simulink model "Ex_xyz"  (R2017b)
settings: Solver=VariableStepAuto  StartTime=0.0  StopTime=1  RelTol=1e-3
settings Model: Creator=81068  LastModifiedBy=81068

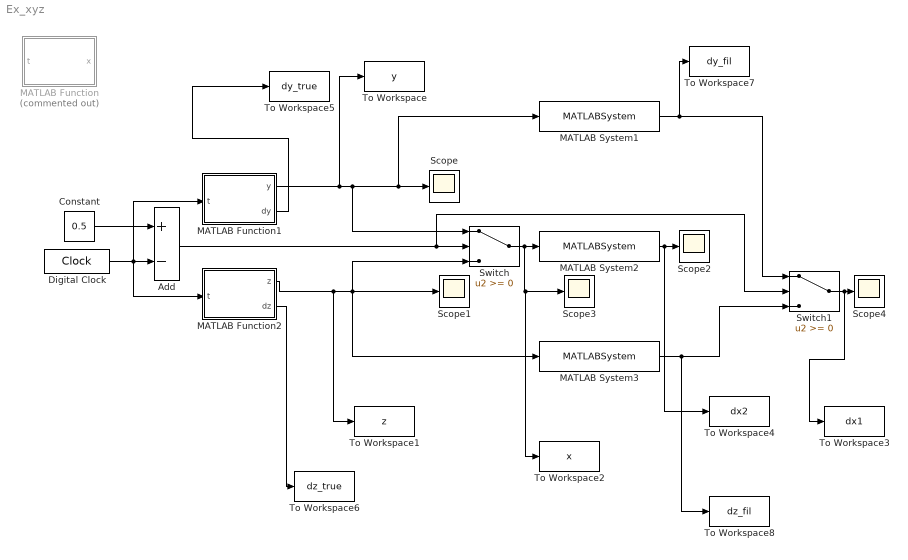
== system Ex_xyz ==
  Add : Sum  Inputs=+-
  Constant : Constant  Value=0.5
  Digital Clock : DigitalClock  SampleTime=1/2000
  MATLAB Function : MATLAB Function  Commented=on  TreatAsAtomicUnit=on
  MATLAB Function1 : MATLAB Function  TreatAsAtomicUnit=on
  MATLAB Function2 : MATLAB Function  TreatAsAtomicUnit=on
  MATLAB System1 : MATLABSystem  System=PolyRegressionFilter  sample_time=1/2000  history_length=10  dop=1  signal_dim=1  delay=RegressionDelay  SimulateUsing=Code generation
      mask Type: PolyRegressionFilter
      mask Display:
      | disp('PolyRegressionFilter');
      | port_label('input',1,'q');
      | port_label('output',1,'dq');
  MATLAB System2 : MATLABSystem  System=PolyRegressionFilter  sample_time=1/2000  history_length=10  dop=1  signal_dim=1  delay=RegressionDelay  SimulateUsing=Code generation
      mask Type: PolyRegressionFilter
      mask Display:
      | disp('PolyRegressionFilter');
      | port_label('input',1,'q');
      | port_label('output',1,'dq');
  MATLAB System3 : MATLABSystem  System=PolyRegressionFilter  sample_time=1/2000  history_length=10  dop=1  signal_dim=1  delay=RegressionDelay  SimulateUsing=Code generation
      mask Type: PolyRegressionFilter
      mask Display:
      | disp('PolyRegressionFilter');
      | port_label('input',1,'q');
      | port_label('output',1,'dq');
  Scope{,1..4} (5 alike) : Scope
  Switch : Switch
  Switch1 : Switch
  To Workspace : ToWorkspace  VariableName=y  SaveFormat=Timeseries  SampleTime=-1
  To Workspace1 : ToWorkspace  VariableName=z  SaveFormat=Timeseries  SampleTime=-1
  To Workspace2 : ToWorkspace  VariableName=x  SaveFormat=Timeseries  SampleTime=-1
  To Workspace3 : ToWorkspace  VariableName=dx1  SaveFormat=Timeseries  SampleTime=-1
  To Workspace4 : ToWorkspace  VariableName=dx2  SaveFormat=Timeseries  SampleTime=-1
  To Workspace5 : ToWorkspace  VariableName=dy_true  SaveFormat=Timeseries  SampleTime=-1
  To Workspace6 : ToWorkspace  VariableName=dz_true  SaveFormat=Timeseries  SampleTime=-1
  To Workspace7 : ToWorkspace  VariableName=dy_fil  SaveFormat=Timeseries  SampleTime=-1
  To Workspace8 : ToWorkspace  VariableName=dz_fil  SaveFormat=Timeseries  SampleTime=-1
  wires:
  Constant/1 -> Add/1
  Digital Clock/1 -> MATLAB Function2/1(t), MATLAB Function1/1(t), Add/2
  Add/1 -> Switch1/2, Switch/2
  MATLAB Function2/1(z) -> To Workspace1/1, MATLAB System3/1, Scope1/1, Switch/3
  Switch/1 -> To Workspace2/1, Scope3/1, MATLAB System2/1
  MATLAB System2/1 -> To Workspace4/1, Scope2/1
  MATLAB System1/1 -> To Workspace7/1, Switch1/1
  MATLAB System3/1 -> To Workspace8/1, Switch1/3
  Switch1/1 -> To Workspace3/1, Scope4/1
  MATLAB Function1/1(y) -> To Workspace/1, Switch/1, MATLAB System1/1, Scope/1
  MATLAB Function1/2(dy) -> To Workspace5/1
  MATLAB Function2/2(dz) -> To Workspace6/1

== matlab function Ex_xyz/MATLAB Function1 ==
  data: t input; y output; dy output
function [y,dy] = fcn(t)
a = 16;
if t<0.5
    y = t;
    dy = 1;
else
    y = a*(t-0.75)^2 + t - 0.25^2*a;
    dy = 2*a*(t-0.75) + 1;
end

== matlab function Ex_xyz/MATLAB Function ==
  data: t input; x output
function x = fcn(t)

x = t;

== matlab function Ex_xyz/MATLAB Function2 ==
  data: t input; z output; dz output
function [z,dz] = fcn(t)

a = 16;
if t<0.5
    z = a*(t-0.25)^2 + t - 0.25^2*a;
    dz = 2*a*(t-0.25)+1;
else
    z = t;
    dz = 1;
end
